simulink model "kensyu_2r_mf"  (R2019a)
settings: Solver=ode4  StartTime=0  StopTime=Analysis_Time  FixedStep=Step_Time  RelTol=1e-3  EnableMultiTasking=on
values from neighbouring files (symbols this model uses):
  a0 = 1.3    [mf.mat]    (also in model_2r.m; model_Fy.m)
  a1 = -0.0274    [mf.mat]    (also in model_2r.m; model_Fy.m)
  a10 = 0.015    [mf.mat]    (also in model_2r.m; model_Fy.m)
  a11 = 0.00849    [mf.mat]    (also in model_2r.m = 0.0849; model_Fy.m)
  a12 = -0.0103    [mf.mat]    (also in model_2r.m; model_Fy.m)
  a13 = 0.0395    [mf.mat]    (also in model_2r.m; model_Fy.m)
  a2 = 1.05    [mf.mat]    (also in model_2r.m; model_Fy.m)
  a3 = 1.18    [mf.mat]    (also in model_2r.m; model_Fy.m)
  a4 = 7.69    [mf.mat]    (also in model_2r.m; model_Fy.m)
  a6 = -0.257    [mf.mat]    (also in model_2r.m; model_Fy.m)
  a7 = 0.224    [mf.mat]    (also in model_2r.m; model_Fy.m)
  a8 = 0.025    [mf.mat]    (also in model_2r.m; model_Fy.m)
  a9 = 0.01    [mf.mat]    (also in model_2r.m; model_Fy.m)
  camber = 0    [model_2r.m]
  g = 9.81    [mf.mat]    (also in model_2r.m)
  Iz = 1500    [mf.mat]    (also in model_2r.m)
  lf = 1.4    [mf.mat]    (also in model_2r.m = 1.2)
  lr = 1.2    [mf.mat]    (also in model_2r.m = 1.4)
  m = 1200    [mf.mat]    (also in model_2r.m)
  V = v/3.6    (= 27.7777777778)    [model_2r.m]
libraries: simulink_extras x10, simulink x1
settings Model: Creator=Iwasaki  LastModifiedBy=katsu
settings DataIOCC: LimitDataPoints=on  SaveFormat=Array  ReturnWorkspaceOutputs=off
settings OptimizationCC: LifeSpan=inf
settings DebuggingCC: UnderspecifiedInitializationDetection=Classic  MergeDetectMultiDrivingBlocksExec=none  SolverPrmCheckMsg=warning  SFUnexpectedBacktrackingDiag=warning  SFNoUnconditionalDefaultTransitionDiag=warning  SFExecutionAtInitializationDiag=none  ArithmeticOperatorsInVariantConditions=warning
settings HardwareCC: ProdBitPerPointer=32  ProdBitPerSizeT=32  ProdBitPerPtrDiffT=32  ProdLargestAtomicFloat=None  ProdIntDivRoundTo=Undefined  ProdEndianess=Unspecified  ProdWordSize=32  ProdHWDeviceType=32-bit Generic
settings ModelReferenceCC: PropagateSignalLabelsOutOfModel=off
settings SFSimCC: SimUseLocalCustomCode=off
settings RTWCC: RTWUseLocalCustomCode=off
settings CodeAppCC: StateflowObjectComments=on
settings GRTTargetCC: TargetLangStandard=C89/C90 (ANSI)  GeneratePreprocessorConditionals=Disable all
settings ConfigComp: CovMetricSettings=dw  CovHtmlReporting=on  CovSaveCumulativeToWorkspaceVar=on  CovSaveSingleToWorkspaceVar=on  CovExternalEMLEnable=off

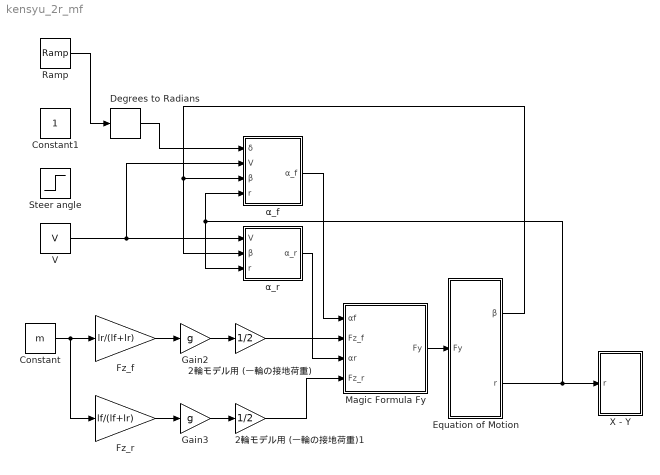
== system kensyu_2r_mf ==
  2輪モデル用 (一輪の接地荷重) : Gain  Gain=1/2
  2輪モデル用 (一輪の接地荷重)1 : Gain  Gain=1/2
  Constant : Constant  Value=m
  Constant1 : Constant
  Degrees to Radians : simulink_extras/Transformations/Degrees to Radians
  Equation of Motion : Subsystem
  Fz_f : Gain  Gain=lr/(lf+lr)
  Fz_r : Gain  Gain=lf/(lf+lr)
  Gain2 : Gain  Gain=g
  Gain3 : Gain  Gain=g
  Magic Formula Fy : Subsystem
  Ramp : simulink/Sources/Ramp  slope=1  start=0  InitialOutput=0
  Steer angle : Step  SampleTime=0
  V : Constant  Value=V
  X - Y : Subsystem
  α_f : Subsystem
  α_r : Subsystem
  wires:
  Magic Formula Fy/1(Fy) -> Equation of Motion/1(Fy)
  Constant/1 -> Fz_f/1, Fz_r/1
  Fz_f/1 -> Gain2/1
  Fz_r/1 -> Gain3/1
  2輪モデル用 (一輪の接地荷重)/1 -> Magic Formula Fy/2(Fz_f)
  2輪モデル用 (一輪の接地荷重)1/1 -> Magic Formula Fy/4(Fz_r)
  Gain2/1 -> 2輪モデル用 (一輪の接地荷重)/1
  Gain3/1 -> 2輪モデル用 (一輪の接地荷重)1/1
  Equation of Motion/2(r) -> α_r/3(r), α_f/4(r), X - Y/1(r)
  Degrees to Radians/1 -> α_f/1(δ)
  V/1 -> α_r/1(V), α_f/2(V)
  α_f/1(α_f) -> Magic Formula Fy/1(αf)
  α_r/1(α_r) -> Magic Formula Fy/3(αr)
  Equation of Motion/1(β) -> α_f/3(β), α_r/2(β)
  Ramp/1 -> Degrees to Radians/1

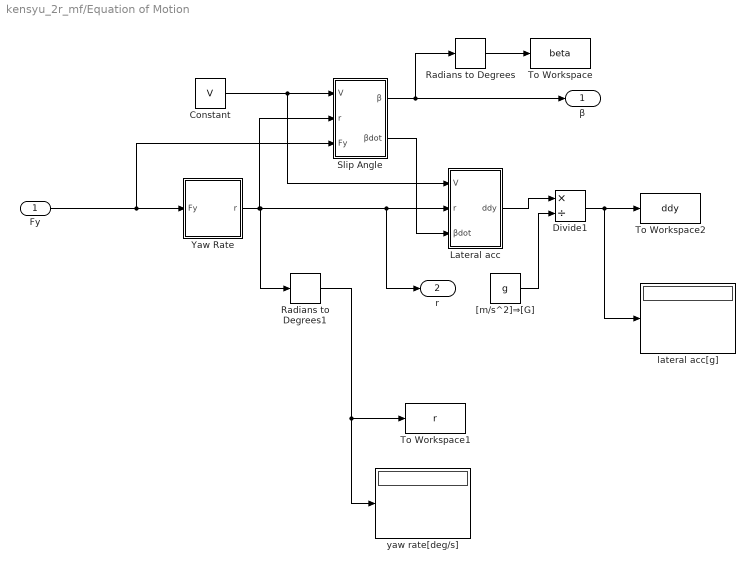
== system kensyu_2r_mf/Equation of Motion ==
  Fy : Inport
  Constant : Constant  Value=V
  Divide1 : Product  Inputs=*/
  Lateral acc : Subsystem
  Radians to Degrees : simulink_extras/Transformations/Radians to Degrees
  Radians to Degrees1 : simulink_extras/Transformations/Radians to Degrees
  Slip Angle : Subsystem
  To Workspace : ToWorkspace  VariableName=beta  SampleTime=-1
  To Workspace1 : ToWorkspace  VariableName=r  SampleTime=-1
  To Workspace2 : ToWorkspace  VariableName=ddy  SampleTime=-1
  Yaw Rate : Subsystem
  "[m/s^2]⇒[G]" : Constant  Value=g
  lateral acc[g] : Display
  yaw rate[deg/s] : Display
  β : Outport
  r : Outport  Port=2
  wires:
  Radians to Degrees/1 -> To Workspace/1
  Radians to Degrees1/1 -> yaw rate[deg/s]/1, To Workspace1/1
  Fy/1 -> Slip Angle/3(Fy), Yaw Rate/1("Fy ")
  Slip Angle/1(β) -> β/1, Radians to Degrees/1
  Yaw Rate/1(r) -> Lateral acc/2(r), r/1, Radians to Degrees1/1, Slip Angle/2(r)
  Constant/1 -> Lateral acc/1(V), Slip Angle/1(V)
  "[m/s^2]⇒[G]"/1 -> Divide1/2
  Divide1/1 -> lateral acc[g]/1, To Workspace2/1
  Lateral acc/1(ddy) -> Divide1/1
  Slip Angle/2(βdot) -> Lateral acc/3(βdot)

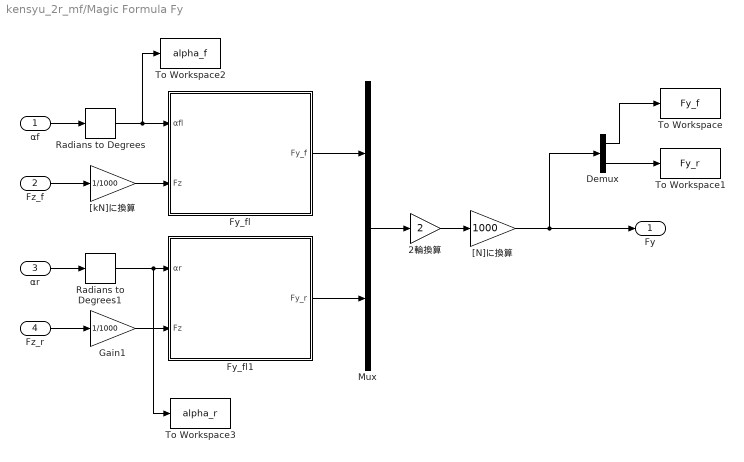
== system kensyu_2r_mf/Magic Formula Fy ==
  αf : Inport
  Fz_f : Inport  Port=2
  αr : Inport  Port=3
  Fz_r : Inport  Port=4
  2輪換算 : Gain  Gain=2
  Demux : Demux  Outputs=2
  Fy_fl : Subsystem
  Fy_fl1 : Subsystem
  Gain1 : Gain  Gain=1/1000
  Mux : Mux  Inputs=2
  Radians to Degrees : simulink_extras/Transformations/Radians to Degrees
  Radians to Degrees1 : simulink_extras/Transformations/Radians to Degrees
  To Workspace : ToWorkspace  VariableName=Fy_f  SampleTime=-1
  To Workspace1 : ToWorkspace  VariableName=Fy_r  SampleTime=-1
  To Workspace2 : ToWorkspace  VariableName=alpha_f  SampleTime=-1
  To Workspace3 : ToWorkspace  VariableName=alpha_r  SampleTime=-1
  "[N]に換算" : Gain  Gain=1000
  "[kN]に換算" : Gain  Gain=1/1000
  Fy : Outport
  wires:
  Mux/1 -> 2輪換算/1
  Fz_f/1 -> "[kN]に換算"/1
  Fz_r/1 -> Gain1/1
  Fy_fl/1(Fy_f) -> Mux/1
  Fy_fl1/1(Fy_r) -> Mux/2
  2輪換算/1 -> "[N]に換算"/1
  αf/1 -> Radians to Degrees/1
  αr/1 -> Radians to Degrees1/1
  "[kN]に換算"/1 -> Fy_fl/2(Fz)
  Gain1/1 -> Fy_fl1/2(Fz)
  Demux/1 -> To Workspace/1
  Demux/2 -> To Workspace1/1
  Radians to Degrees/1 -> To Workspace2/1, Fy_fl/1(αfl)
  "[N]に換算"/1 -> Fy/1, Demux/1
  Radians to Degrees1/1 -> To Workspace3/1, Fy_fl1/1(αr)

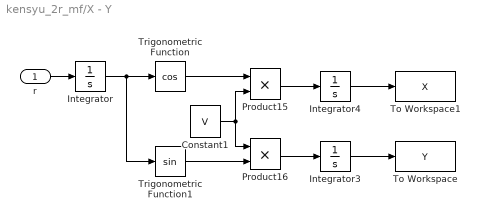
== system kensyu_2r_mf/X - Y ==
  r : Inport
  Constant1 : Constant  Value=V
  Integrator : Integrator
  Integrator3 : Integrator
  Integrator4 : Integrator
  Product15 : Product  RndMeth=Zero
  Product16 : Product  RndMeth=Zero
  To Workspace : ToWorkspace  VariableName=Y  SampleTime=-1
  To Workspace1 : ToWorkspace  VariableName=X  SampleTime=-1
  Trigonometric Function : Trigonometry  Operator=cos
  Trigonometric Function1 : Trigonometry
  wires:
  Product16/1 -> Integrator3/1
  Integrator4/1 -> To Workspace1/1
  Product15/1 -> Integrator4/1
  Integrator3/1 -> To Workspace/1
  Trigonometric Function/1 -> Product15/1
  r/1 -> Integrator/1
  Constant1/1 -> Product15/2, Product16/1
  Trigonometric Function1/1 -> Product16/2
  Integrator/1 -> Trigonometric Function1/1, Trigonometric Function/1

== system kensyu_2r_mf/α_f ==
  δ : Inport
  V : Inport  Port=2
  β : Inport  Port=3
  r : Inport  Port=4
  Constant : Constant  Value=lf
  Divide : Product  Inputs=**
  Divide1 : Product  Inputs=*/
  Subtract2 : Sum  Inputs=+--
  α_f : Outport
  wires:
  δ/1 -> Subtract2/1
  β/1 -> Subtract2/2
  Divide/1 -> Divide1/1
  r/1 -> Divide/2
  Constant/1 -> Divide/1
  V/1 -> Divide1/2
  Divide1/1 -> Subtract2/3
  Subtract2/1 -> α_f/1

== system kensyu_2r_mf/α_r ==
  V : Inport
  β : Inport  Port=2
  r : Inport  Port=3
  Add : Sum  Inputs=-+
  Constant : Constant  Value=lr
  Divide : Product  Inputs=**
  Divide1 : Product  Inputs=*/
  α_r : Outport
  wires:
  β/1 -> Add/1
  Constant/1 -> Divide/1
  r/1 -> Divide/2
  Divide/1 -> Divide1/1
  V/1 -> Divide1/2
  Divide1/1 -> Add/2
  Add/1 -> α_r/1

== system kensyu_2r_mf/Equation of Motion/Lateral acc ==
  V : Inport
  r : Inport  Port=2
  βdot : Inport  Port=3
  Add : Sum
  Divide : Product  Inputs=**
  ddy : Outport
  wires:
  r/1 -> Add/1
  βdot/1 -> Add/2
  V/1 -> Divide/1
  Add/1 -> Divide/2
  Divide/1 -> ddy/1

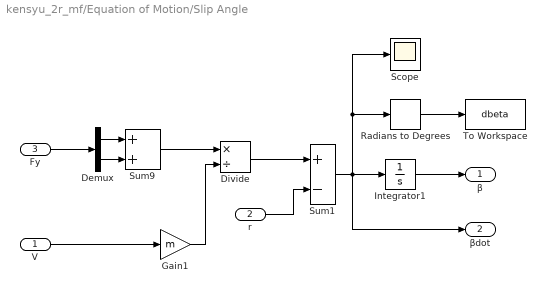
== system kensyu_2r_mf/Equation of Motion/Slip Angle ==
  V : Inport
  r : Inport  Port=2
  Fy : Inport  Port=3
  Demux : Demux  Outputs=2
  Divide : Product  Inputs=*/
  Gain1 : Gain  Gain=m
  Integrator1 : Integrator
  Radians to Degrees : simulink_extras/Transformations/Radians to Degrees
  Scope : Scope
  Sum1 : Sum  Inputs=+-
  Sum9 : Sum
  To Workspace : ToWorkspace  VariableName=dbeta  SampleTime=-1
  β : Outport
  βdot : Outport  Port=2
  wires:
  V/1 -> Gain1/1
  Sum9/1 -> Divide/1
  Divide/1 -> Sum1/1
  r/1 -> Sum1/2
  Sum1/1 -> βdot/1, Integrator1/1, Scope/1, Radians to Degrees/1
  Fy/1 -> Demux/1
  Demux/2 -> Sum9/2
  Demux/1 -> Sum9/1
  Integrator1/1 -> β/1
  Gain1/1 -> Divide/2
  Radians to Degrees/1 -> To Workspace/1

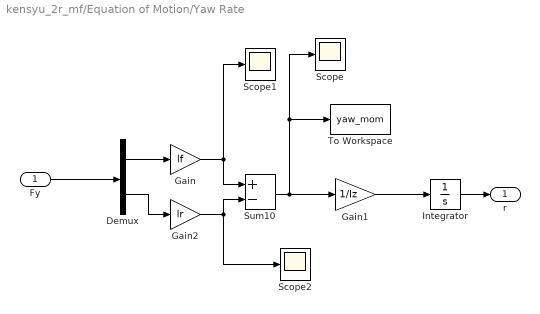
== system kensyu_2r_mf/Equation of Motion/Yaw Rate ==
  "Fy " : Inport
  Demux : Demux  Outputs=2
  Gain : Gain  Gain=lf
  Gain1 : Gain  Gain=1/Iz
  Gain2 : Gain  Gain=lr
  Integrator : Integrator
  Scope : Scope
  Scope1 : Scope
  Scope2 : Scope
  Sum10 : Sum  Inputs=+-
  To Workspace : ToWorkspace  VariableName=yaw_mom  SampleTime=-1
  r : Outport
  wires:
  Gain1/1 -> Integrator/1
  Sum10/1 -> Scope/1, To Workspace/1, Gain1/1
  Demux/2 -> Gain2/1
  Demux/1 -> Gain/1
  Gain/1 -> Sum10/1, Scope1/1
  Gain2/1 -> Scope2/1, Sum10/2
  "Fy "/1 -> Demux/1
  Integrator/1 -> r/1

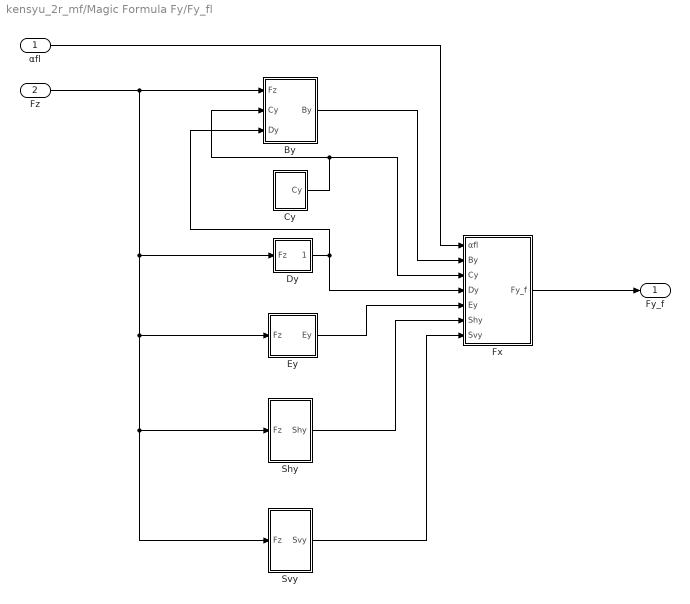
== system kensyu_2r_mf/Magic Formula Fy/Fy_fl ==
  αfl : Inport
  Fz : Inport  Port=2
  By : Subsystem
  Cy : Subsystem
  Dy : Subsystem
  Ey : Subsystem
  Fx : Subsystem
  Shy : Subsystem
  Svy : Subsystem
  Fy_f : Outport
  wires:
  Dy/1(Dy) -> Fx/4(Dy), By/3(Dy)
  Cy/1(Cy) -> Fx/3(Cy), By/2(Cy)
  By/1(By) -> Fx/2(By)
  αfl/1 -> Fx/1(αfl)
  Shy/1(Shy) -> Fx/6(Shy)
  Ey/1(Ey) -> Fx/5(Ey)
  Svy/1(Svy) -> Fx/7(Svy)
  Fz/1 -> Ey/1(Fz), Svy/1(Fz), Shy/1(Fz), Dy/1(Fz), By/1(Fz)
  Fx/1(Fy_f) -> Fy_f/1

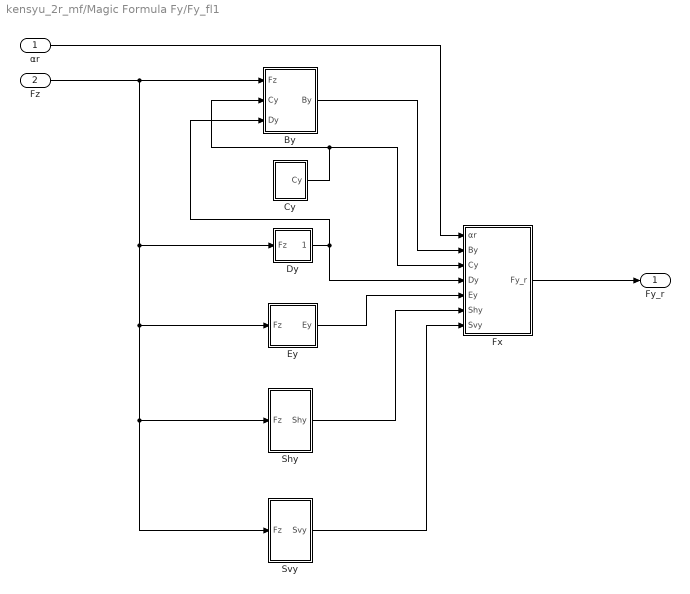
== system kensyu_2r_mf/Magic Formula Fy/Fy_fl1 ==
  αr : Inport
  Fz : Inport  Port=2
  By : Subsystem
  Cy : Subsystem
  Dy : Subsystem
  Ey : Subsystem
  Fx : Subsystem
  Shy : Subsystem
  Svy : Subsystem
  Fy_r : Outport
  wires:
  Dy/1(Dy) -> Fx/4(Dy), By/3(Dy)
  Cy/1(Cy) -> Fx/3(Cy), By/2(Cy)
  By/1(By) -> Fx/2(By)
  αr/1 -> Fx/1(αr)
  Shy/1(Shy) -> Fx/6(Shy)
  Ey/1(Ey) -> Fx/5(Ey)
  Svy/1(Svy) -> Fx/7(Svy)
  Fz/1 -> Ey/1(Fz), Svy/1(Fz), Shy/1(Fz), Dy/1(Fz), By/1(Fz)
  Fx/1(Fy_r) -> Fy_r/1

== system kensyu_2r_mf/Magic Formula Fy/Fy_fl/By ==
  Fz : Inport
  Cy : Inport  Port=2
  Dy : Inport  Port=3
  BCDy : Subsystem
  Divide : Product  Inputs=*/
  Product : Product
  By : Outport
  wires:
  BCDy/1(BCDy) -> Divide/1
  Product/1 -> Divide/2
  Dy/1 -> Product/1
  Cy/1 -> Product/2
  Divide/1 -> By/1
  Fz/1 -> BCDy/1(Fz)

== system kensyu_2r_mf/Magic Formula Fy/Fy_fl/Cy ==
  Constant : Constant  Value=a0
  Cy : Outport
  wires:
  Constant/1 -> Cy/1

== system kensyu_2r_mf/Magic Formula Fy/Fy_fl/Dy ==
  Fz : Inport
  Product : Product
  μy : Subsystem
  Dy : Outport
  wires:
  Product/1 -> Dy/1
  μy/1(μy) -> Product/2
  Fz/1 -> μy/1(Fz), Product/1

== system kensyu_2r_mf/Magic Formula Fy/Fy_fl/Ey ==
  Fz : Inport
  Constant : Constant  Value=a6
  Constant1 : Constant  Value=a7
  Product : Product
  Subtract : Sum
  Ey : Outport
  wires:
  Subtract/1 -> Ey/1
  Fz/1 -> Product/1
  Constant/1 -> Product/2
  Constant1/1 -> Subtract/2
  Product/1 -> Subtract/1

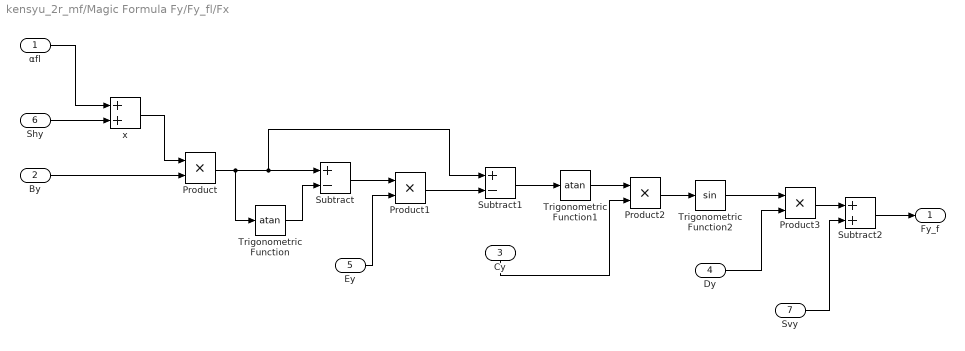
== system kensyu_2r_mf/Magic Formula Fy/Fy_fl/Fx ==
  αfl : Inport
  By : Inport  Port=2
  Cy : Inport  Port=3
  Dy : Inport  Port=4
  Ey : Inport  Port=5
  Shy : Inport  Port=6
  Svy : Inport  Port=7
  Product{,1..3} (4 alike) : Product
  Subtract : Sum  Inputs=+-
  Subtract1 : Sum  Inputs=+-
  Subtract2 : Sum
  Trigonometric Function : Trigonometry  Operator=atan
  Trigonometric Function1 : Trigonometry  Operator=atan
  Trigonometric Function2 : Trigonometry
  x : Sum
  Fy_f : Outport
  wires:
  Subtract2/1 -> Fy_f/1
  Dy/1 -> Product3/2
  Cy/1 -> Product2/2
  Product2/1 -> Trigonometric Function2/1
  x/1 -> Product/1
  Trigonometric Function1/1 -> Product2/1
  Subtract1/1 -> Trigonometric Function1/1
  Trigonometric Function2/1 -> Product3/1
  Svy/1 -> Subtract2/2
  Ey/1 -> Product1/2
  αfl/1 -> x/1
  By/1 -> Product/2
  Shy/1 -> x/2
  Product3/1 -> Subtract2/1
  Trigonometric Function/1 -> Subtract/2
  Product1/1 -> Subtract1/2
  Product/1 -> Trigonometric Function/1, Subtract1/1, Subtract/1
  Subtract/1 -> Product1/1

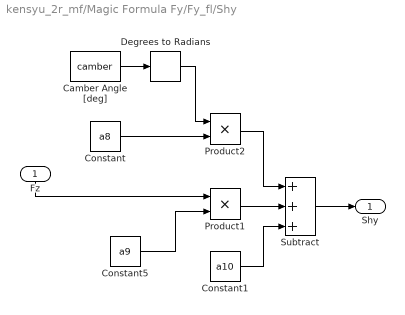
== system kensyu_2r_mf/Magic Formula Fy/Fy_fl/Shy ==
  Fz : Inport
  Camber Angle [deg] : Constant  Value=camber
  Constant : Constant  Value=a8
  Constant1 : Constant  Value=a10
  Constant5 : Constant  Value=a9
  Degrees to Radians : simulink_extras/Transformations/Degrees to Radians
  Product1 : Product
  Product2 : Product
  Subtract : Sum  Inputs=+++
  Shy : Outport
  wires:
  Constant5/1 -> Product1/2
  Fz/1 -> Product1/1
  Subtract/1 -> Shy/1
  Constant1/1 -> Subtract/3
  Product1/1 -> Subtract/2
  Constant/1 -> Product2/2
  Camber Angle [deg]/1 -> Degrees to Radians/1
  Degrees to Radians/1 -> Product2/1
  Product2/1 -> Subtract/1

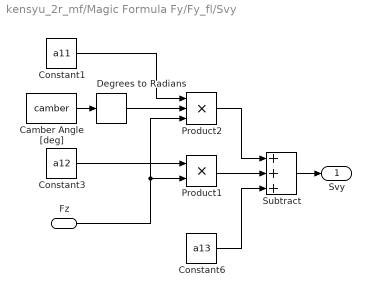
== system kensyu_2r_mf/Magic Formula Fy/Fy_fl/Svy ==
  Fz : Inport
  Camber Angle [deg] : Constant  Value=camber
  Constant1 : Constant  Value=a11
  Constant3 : Constant  Value=a12
  Constant6 : Constant  Value=a13
  Degrees to Radians : simulink_extras/Transformations/Degrees to Radians
  Product1 : Product
  Product2 : Product  Inputs=3
  Subtract : Sum  Inputs=+++
  Svy : Outport
  wires:
  Constant3/1 -> Product1/1
  Subtract/1 -> Svy/1
  Fz/1 -> Product1/2, Product2/3
  Constant6/1 -> Subtract/3
  Product1/1 -> Subtract/2
  Product2/1 -> Subtract/1
  Camber Angle [deg]/1 -> Degrees to Radians/1
  Degrees to Radians/1 -> Product2/2
  Constant1/1 -> Product2/1

== system kensyu_2r_mf/Magic Formula Fy/Fy_fl1/By ==
  Fz : Inport
  Cy : Inport  Port=2
  Dy : Inport  Port=3
  BCDy : Subsystem
  Divide : Product  Inputs=*/
  Product : Product
  By : Outport
  wires:
  BCDy/1(BCDy) -> Divide/1
  Product/1 -> Divide/2
  Dy/1 -> Product/1
  Cy/1 -> Product/2
  Divide/1 -> By/1
  Fz/1 -> BCDy/1(Fz)

== system kensyu_2r_mf/Magic Formula Fy/Fy_fl1/Cy ==
  Constant : Constant  Value=a0
  Cy : Outport
  wires:
  Constant/1 -> Cy/1

== system kensyu_2r_mf/Magic Formula Fy/Fy_fl1/Dy ==
  Fz : Inport
  Product : Product
  μy : Subsystem
  Dy : Outport
  wires:
  Product/1 -> Dy/1
  μy/1(μy) -> Product/2
  Fz/1 -> μy/1(Fz), Product/1

== system kensyu_2r_mf/Magic Formula Fy/Fy_fl1/Ey ==
  Fz : Inport
  Constant : Constant  Value=a6
  Constant1 : Constant  Value=a7
  Product : Product
  Subtract : Sum
  Ey : Outport
  wires:
  Subtract/1 -> Ey/1
  Fz/1 -> Product/1
  Constant/1 -> Product/2
  Constant1/1 -> Subtract/2
  Product/1 -> Subtract/1

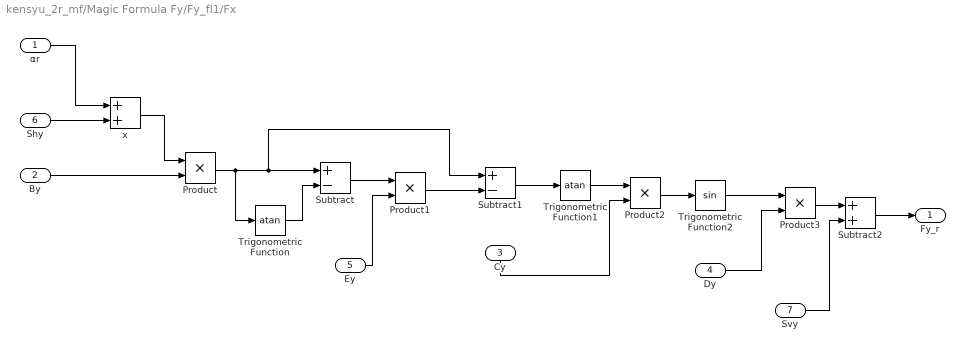
== system kensyu_2r_mf/Magic Formula Fy/Fy_fl1/Fx ==
  αr : Inport
  By : Inport  Port=2
  Cy : Inport  Port=3
  Dy : Inport  Port=4
  Ey : Inport  Port=5
  Shy : Inport  Port=6
  Svy : Inport  Port=7
  Product{,1..3} (4 alike) : Product
  Subtract : Sum  Inputs=+-
  Subtract1 : Sum  Inputs=+-
  Subtract2 : Sum
  Trigonometric Function : Trigonometry  Operator=atan
  Trigonometric Function1 : Trigonometry  Operator=atan
  Trigonometric Function2 : Trigonometry
  x : Sum
  Fy_r : Outport
  wires:
  Subtract2/1 -> Fy_r/1
  Dy/1 -> Product3/2
  Cy/1 -> Product2/2
  Product2/1 -> Trigonometric Function2/1
  x/1 -> Product/1
  Trigonometric Function1/1 -> Product2/1
  Subtract1/1 -> Trigonometric Function1/1
  Trigonometric Function2/1 -> Product3/1
  Svy/1 -> Subtract2/2
  Ey/1 -> Product1/2
  αr/1 -> x/1
  By/1 -> Product/2
  Shy/1 -> x/2
  Product3/1 -> Subtract2/1
  Trigonometric Function/1 -> Subtract/2
  Product1/1 -> Subtract1/2
  Product/1 -> Trigonometric Function/1, Subtract1/1, Subtract/1
  Subtract/1 -> Product1/1

== system kensyu_2r_mf/Magic Formula Fy/Fy_fl1/Shy ==
  Fz : Inport
  Camber Angle [deg] : Constant  Value=camber
  Constant : Constant  Value=a8
  Constant1 : Constant  Value=a10
  Constant5 : Constant  Value=a9
  Degrees to Radians : simulink_extras/Transformations/Degrees to Radians
  Product1 : Product
  Product2 : Product
  Subtract : Sum  Inputs=+++
  Shy : Outport
  wires:
  Constant5/1 -> Product1/2
  Fz/1 -> Product1/1
  Subtract/1 -> Shy/1
  Constant1/1 -> Subtract/3
  Product1/1 -> Subtract/2
  Constant/1 -> Product2/2
  Camber Angle [deg]/1 -> Degrees to Radians/1
  Degrees to Radians/1 -> Product2/1
  Product2/1 -> Subtract/1

== system kensyu_2r_mf/Magic Formula Fy/Fy_fl1/Svy ==
  Fz : Inport
  Camber Angle [deg] : Constant  Value=camber
  Constant1 : Constant  Value=a11
  Constant3 : Constant  Value=a12
  Constant6 : Constant  Value=a13
  Degrees to Radians : simulink_extras/Transformations/Degrees to Radians
  Product1 : Product
  Product2 : Product  Inputs=3
  Subtract : Sum  Inputs=+++
  Svy : Outport
  wires:
  Constant3/1 -> Product1/1
  Subtract/1 -> Svy/1
  Fz/1 -> Product1/2, Product2/3
  Constant6/1 -> Subtract/3
  Product1/1 -> Subtract/2
  Product2/1 -> Subtract/1
  Camber Angle [deg]/1 -> Degrees to Radians/1
  Degrees to Radians/1 -> Product2/2
  Constant1/1 -> Product2/1

== system kensyu_2r_mf/Magic Formula Fy/Fy_fl/By/BCDy ==
  Fz : Inport
  Constant : Constant  Value=a3
  Constant1 : Constant  Value=a4
  Divide : Product  Inputs=*/
  Gain : Gain  Gain=2
  Product2 : Product
  Trigonometric Function : Trigonometry  Operator=atan
  Trigonometric Function1 : Trigonometry
  BCDy : Outport
  wires:
  Trigonometric Function1/1 -> Product2/2
  Divide/1 -> Trigonometric Function/1
  Fz/1 -> Divide/1
  Constant/1 -> Product2/1
  Constant1/1 -> Divide/2
  Trigonometric Function/1 -> Gain/1
  Gain/1 -> Trigonometric Function1/1
  Product2/1 -> BCDy/1

== system kensyu_2r_mf/Magic Formula Fy/Fy_fl/Dy/μy ==
  Fz : Inport
  Constant : Constant  Value=a1
  Constant1 : Constant  Value=a2
  Product : Product
  Subtract : Sum
  μy : Outport
  wires:
  Fz/1 -> Product/1
  Product/1 -> Subtract/1
  Constant/1 -> Product/2
  Constant1/1 -> Subtract/2
  Subtract/1 -> μy/1

== system kensyu_2r_mf/Magic Formula Fy/Fy_fl1/By/BCDy ==
  Fz : Inport
  Constant : Constant  Value=a3
  Constant1 : Constant  Value=a4
  Divide : Product  Inputs=*/
  Gain : Gain  Gain=2
  Product2 : Product
  Trigonometric Function : Trigonometry  Operator=atan
  Trigonometric Function1 : Trigonometry
  BCDy : Outport
  wires:
  Trigonometric Function1/1 -> Product2/2
  Divide/1 -> Trigonometric Function/1
  Fz/1 -> Divide/1
  Constant/1 -> Product2/1
  Constant1/1 -> Divide/2
  Trigonometric Function/1 -> Gain/1
  Gain/1 -> Trigonometric Function1/1
  Product2/1 -> BCDy/1

== system kensyu_2r_mf/Magic Formula Fy/Fy_fl1/Dy/μy ==
  Fz : Inport
  Constant : Constant  Value=a1
  Constant1 : Constant  Value=a2
  Product : Product
  Subtract : Sum
  μy : Outport
  wires:
  Fz/1 -> Product/1
  Product/1 -> Subtract/1
  Constant/1 -> Product/2
  Constant1/1 -> Subtract/2
  Subtract/1 -> μy/1
